simulink model "IMUdataFinalr2PDs"  (R2024a)
settings: Solver=FixedStepAuto  StartTime=0.0  StopTime=100  FixedStep=.01  RelTol=1e-3  EnableMultiTasking=on
undefined symbols (not defined in the file or in its folder): CR, LF
libraries: slpidlib x3, instrumentseriallib x3, hdlsllib x1
settings Model: ExtModeTrigDuration=2  Creator=juanandrespelaezb  LastModifiedBy=Spencer
settings SolverCC: AutoInsertRateTranBlk=on
settings OptimizationCC: EnhancedBackFolding=on  PassReuseOutputArgsThreshold=0  MaxStackSize=64  OptimizeBlockOrder=speed  DifferentSizesBufferReuse=on  OptimizationCustomize=off
settings DebuggingCC: ParameterTunabilityLossMsg=error
settings HardwareCC: ProdBitPerInt=16  ProdBitPerPointer=16  ProdBitPerSizeT=16  ProdBitPerPtrDiffT=16  ProdLargestAtomicFloat=None  ProdWordSize=8  ProdHWDeviceType=Atmel->AVR  UseEmbeddedCoderFeatures=off  UseSimulinkCoderFeatures=off
settings SFSimCC: MATLABDynamicMemAlloc=off
settings RTWCC: Description=Embedded Coder  SystemTargetFile=ert.tlc  HardwareBoard=Arduino Mega 2560  TemplateMakefile=ert_default_tmf  Toolchain=Arduino AVR  BuildConfiguration=Faster Runs
settings CodeAppCC: ForceParamTrailComments=on  OperatorAnnotations=on
settings ERTTargetCC: ERTCustomFileBanners=off  SupportContinuousTime=on  SupportNonInlinedSFcns=on  RemoveResetFunc=off  SupportVariableSizeSignals=on  ModelStepFunctionPrototypeControlCompliant=off  ExtModeTransport=3  ExtModeStaticAlloc=on  ExtModeAutomaticAllocSize=off  ExtModeStaticAllocSize=2048  ExtModeMexFile=ext_xcp  ExtModeIntrfLevel=Level2 - Open

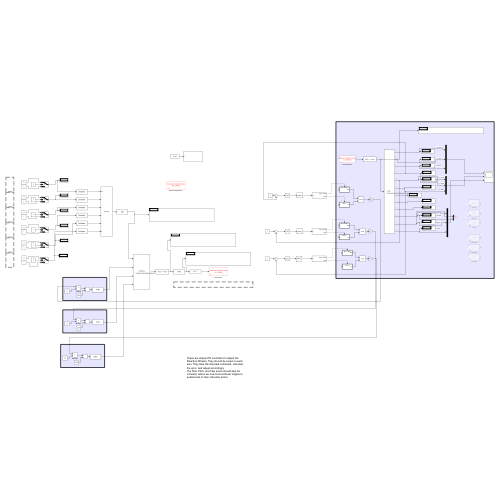
[thumbnail: Simulink's stored preview of the top-level diagram]
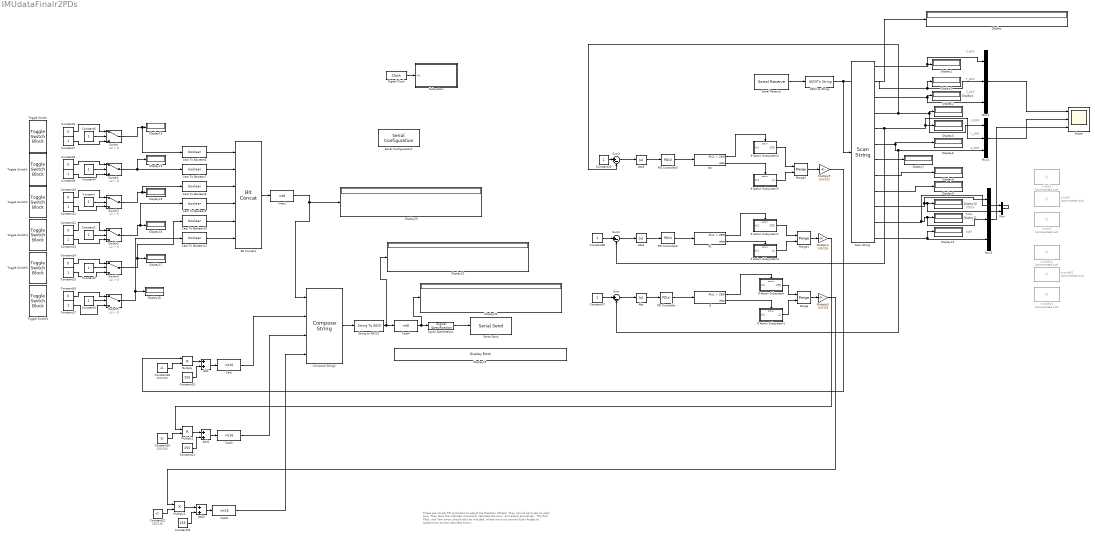
== system IMUdataFinalr2PDs ==
  note: These are simple PD controllers to adjust the Reaction Wheels. They should be tuned on each axis. They take the intended command, calculate the error, and adjust accordingly.
      | The Roll, Pitch, and Yaw errors should also be included, where we must convert Euler Angles to quaternions to then calculate errors.
  note: ROLL
  note: Z_GYR
  note: PITCH
  note: YAW
  note: Y_GYR
  note: X_GYR
  note: Z_ACC
  note: Y_ACC
  note: X_ACC
  ASCII to String : ASCIIToString
  Abs : Abs  SaturateOnIntegerOverflow=off
  Abs2 : Abs  SaturateOnIntegerOverflow=off
  Abs3 : Abs  SaturateOnIntegerOverflow=off
  Add : Sum
  Add1 : Sum
  Add2 : Sum
  Bit Concat1 : hdlsllib/Logic and Bit Operations/Bit Concat  numInputs=6
  Cast : DataTypeConversion  OutDataTypeStr=int16  SaturateOnIntegerOverflow=off  RndMeth=Floor
  Cast To Boolean{6..11} (6 alike) : DataTypeConversion  OutDataTypeStr=boolean  SaturateOnIntegerOverflow=off  RndMeth=Floor
  Cast1 : DataTypeConversion  OutDataTypeStr=int8  SaturateOnIntegerOverflow=off  RndMeth=Floor
  Cast2 : DataTypeConversion  OutDataTypeStr=int16  SaturateOnIntegerOverflow=off  RndMeth=Floor
  Cast3 : DataTypeConversion  OutDataTypeStr=int16  SaturateOnIntegerOverflow=off  RndMeth=Floor
  Cast4 : DataTypeConversion  OutDataTypeStr=int8  SaturateOnIntegerOverflow=off  RndMeth=Floor
  Compose String1 : ComposeString  Format="\"%02d;%03d;%03d;%03d\\n\""
  Constant{,1..5,7,9,11,13,15,17,27..29} (15 alike) : Constant
  Constant{6,8,10,12,14,16} (6 alike) : Constant  Value=0
  Constant18 : Constant  Value=255/100
  Constant19 : Constant  Value=255
  Constant20 : Constant  Value=255/100
  Constant21 : Constant  Value=255
  Constant22 : Constant  Value=255/100
  Constant23 : Constant  Value=255
  Digital Clock : DigitalClock
  Display{,1..18,20..22} (22 alike) : Display
  Display19 : DisplayBlock  LabelPosition=Hide  Format=long  Transparency=1
  If : If  IfExpression=u1 > 255
  If Action Subsystem : Subsystem  TreatAsAtomicUnit=on
  If Action Subsystem1 : Subsystem  TreatAsAtomicUnit=on
  If Action Subsystem2 : Subsystem  TreatAsAtomicUnit=on
  If Action Subsystem3 : Subsystem  TreatAsAtomicUnit=on
  If Action Subsystem4 : Subsystem  TreatAsAtomicUnit=on
  If Action Subsystem5 : Subsystem  TreatAsAtomicUnit=on
  If1 : If  IfExpression=u1 > 255
  If2 : If  IfExpression=u1 > 255
  Merge : Merge
  Merge1 : Merge
  Merge2 : Merge
  Multiply : Product
  Multiply1 : Product
  Multiply2 : Product
  Multiply3 : Gain  Gain=100/255
  Multiply4 : Gain  Gain=100/255
  Multiply5 : Gain  Gain=100/255
  Mux : Mux  Inputs=2
  Mux1 : Mux  Inputs=3
  Mux2 : Mux  Inputs=3
  Mux3 : Mux  Inputs=3
  PID Controller : slpidlib/PID Controller  Controller=PD  Form=Parallel  TimeDomain=Continuous-time  UseExternalTs=off  SampleTime=-1  IntegratorMethod=Forward Euler  FilterMethod=Forward Euler  ControllerParametersSource=internal  P=25  I=1  UseKiTs=off  D=5  UseExternalDerivativeSource=off  N=100  UseFilter=on  TunerSelectOption=Transfer Function Based (PID Tuner App)  InitialConditionSource=internal  InitialConditionForIntegrator=0  InitialConditionForFilter=0  DifferentiatorICPrevScaledInput=0  ExternalReset=none  TrackingMode=off  Kt=1  LimitOutput=off  SatLimitsSource=internal  UpperSaturationLimit=inf  LowerSaturationLimit=-inf  LinearizeAsGain=on  AntiWindupMode=none  Kb=1  LimitIntegrator=off  UpperIntegratorSaturationLimit=inf  LowerIntegratorSaturationLimit=-inf  POutMin=[]  POutMax=[]  IOutMin=[]  IOutMax=[]  DOutMin=[]  DOutMax=[]  NOutMin=[]  NOutMax=[]  SumOutMin=[]  SumOutMax=[]  SaturationOutMin=[]  SaturationOutMax=[]  PParamMin=[]  PParamMax=[]  IParamMin=[]  IParamMax=[]  DParamMin=[]  DParamMax=[]  NParamMin=[]  NParamMax=[]  KbParamMin=[]  KbParamMax=[]  KtParamMin=[]  KtParamMax=[]  KbOutMin=[]  KbOutMax=[]  KtOutMin=[]  KtOutMax=[]  IntegratorOutMin=[]  IntegratorOutMax=[]  FilterOutMin=[]  FilterOutMax=[]  SumI1OutMin=[]  SumI1OutMax=[]  SumI2OutMin=[]  SumI2OutMax=[]  SumI3OutMin=[]  SumI3OutMax=[]  SumI4OutMin=[]  SumI4OutMax=[]  SumDOutMin=[]  SumDOutMax=[]  DifferentiatorOutMin=[]  DifferentiatorOutMax=[]  FilterDiffOutCoefMin=[]  FilterDiffOutCoefMax=[]  ReciprocalOutMin=[]  ReciprocalOutMax=[]  SumDenOutMin=[]  SumDenOutMax=[]  SumNumOutMin=[]  SumNumOutMax=[]  DivideOutMin=[]  DivideOutMax=[]  UdiffTsProdOutMin=[]  UdiffTsProdOutMax=[]  NTsProdOutMin=[]  NTsProdOutMax=[]  UintegralTsProdOutMin=[]  UintegralTsProdOutMax=[]  UngainTsProdOutMin=[]  UngainTsProdOutMax=[]  ClampingZeroOutDataTypeStr=Inherit: Inherit via back propagation  ClampingZeroOutMin=[]  ClampingZeroOutMax=[]  FilterDenConstantOutDataTypeStr=Inherit: Inherit via back propagation  FilterDenConstantOutMin=[]  FilterDenConstantOutMax=[]  PCopyOutDataTypeStr=Inherit: Inherit via back propagation  PCopyOutMin=[]  PCopyOutMax=[]  NCopyOutDataTypeStr=Inherit: Inherit via back propagation  NCopyOutMin=[]  NCopyOutMax=[]  IntegratorContinuousStateAttributes=''  IntegratorStateMustResolveToSignalObject=off  IntegratorRTWStateStorageClass=Auto  FilterContinuousStateAttributes=''  FilterStateMustResolveToSignalObject=off  FilterRTWStateStorageClass=Auto  ParallelPVariant=InternalParameters  IdealPVariant=Disabled  IVariant=Disabled  DVariant=InternalParameters  IntegratorVariant=Disabled  SatVariant=Disabled  AWVariant=Disabled  PCopyVariant=Disabled  TRVariant=Disabled  FdbkBlocksVariant=Forward  IdealPFdbkVariant=Disabled  SatFdbkVariant=Disabled  DerivativeFilterVariant=ContFilter  NVariant=InternalParameters  NCopyVariant=Disabled  FilterICVariant=InternalICsFilter  IntegratorICVariant=Disabled  ExternalResetVariant=Disabled  TRSumVariant=Passthrough  SumFdbkVariant=Disabled  SumVariant=Sum_PD  TsampFilterVariant=InternalTs  TsampNgainVariant=Passthrough  TsampIntegralVariant=Disabled_SignalSpec  ExternalSaturationOutDataTypeStr=Inherit: Same as second input  DerivativeSourceVariant=ErrorSignal
  PID Controller2 : slpidlib/PID Controller  Controller=PD  Form=Parallel  TimeDomain=Continuous-time  UseExternalTs=off  SampleTime=-1  IntegratorMethod=Forward Euler  FilterMethod=Forward Euler  ControllerParametersSource=internal  P=25  I=1  UseKiTs=off  D=5  UseExternalDerivativeSource=off  N=100  UseFilter=on  TunerSelectOption=Transfer Function Based (PID Tuner App)  InitialConditionSource=internal  InitialConditionForIntegrator=0  InitialConditionForFilter=0  DifferentiatorICPrevScaledInput=0  ExternalReset=none  TrackingMode=off  Kt=1  LimitOutput=off  SatLimitsSource=internal  UpperSaturationLimit=inf  LowerSaturationLimit=-inf  LinearizeAsGain=on  AntiWindupMode=none  Kb=1  LimitIntegrator=off  UpperIntegratorSaturationLimit=inf  LowerIntegratorSaturationLimit=-inf  POutMin=[]  POutMax=[]  IOutMin=[]  IOutMax=[]  DOutMin=[]  DOutMax=[]  NOutMin=[]  NOutMax=[]  SumOutMin=[]  SumOutMax=[]  SaturationOutMin=[]  SaturationOutMax=[]  PParamMin=[]  PParamMax=[]  IParamMin=[]  IParamMax=[]  DParamMin=[]  DParamMax=[]  NParamMin=[]  NParamMax=[]  KbParamMin=[]  KbParamMax=[]  KtParamMin=[]  KtParamMax=[]  KbOutMin=[]  KbOutMax=[]  KtOutMin=[]  KtOutMax=[]  IntegratorOutMin=[]  IntegratorOutMax=[]  FilterOutMin=[]  FilterOutMax=[]  SumI1OutMin=[]  SumI1OutMax=[]  SumI2OutMin=[]  SumI2OutMax=[]  SumI3OutMin=[]  SumI3OutMax=[]  SumI4OutMin=[]  SumI4OutMax=[]  SumDOutMin=[]  SumDOutMax=[]  DifferentiatorOutMin=[]  DifferentiatorOutMax=[]  FilterDiffOutCoefMin=[]  FilterDiffOutCoefMax=[]  ReciprocalOutMin=[]  ReciprocalOutMax=[]  SumDenOutMin=[]  SumDenOutMax=[]  SumNumOutMin=[]  SumNumOutMax=[]  DivideOutMin=[]  DivideOutMax=[]  UdiffTsProdOutMin=[]  UdiffTsProdOutMax=[]  NTsProdOutMin=[]  NTsProdOutMax=[]  UintegralTsProdOutMin=[]  UintegralTsProdOutMax=[]  UngainTsProdOutMin=[]  UngainTsProdOutMax=[]  ClampingZeroOutDataTypeStr=Inherit: Inherit via back propagation  ClampingZeroOutMin=[]  ClampingZeroOutMax=[]  FilterDenConstantOutDataTypeStr=Inherit: Inherit via back propagation  FilterDenConstantOutMin=[]  FilterDenConstantOutMax=[]  PCopyOutDataTypeStr=Inherit: Inherit via back propagation  PCopyOutMin=[]  PCopyOutMax=[]  NCopyOutDataTypeStr=Inherit: Inherit via back propagation  NCopyOutMin=[]  NCopyOutMax=[]  IntegratorContinuousStateAttributes=''  IntegratorStateMustResolveToSignalObject=off  IntegratorRTWStateStorageClass=Auto  FilterContinuousStateAttributes=''  FilterStateMustResolveToSignalObject=off  FilterRTWStateStorageClass=Auto  ParallelPVariant=InternalParameters  IdealPVariant=Disabled  IVariant=Disabled  DVariant=InternalParameters  IntegratorVariant=Disabled  SatVariant=Disabled  AWVariant=Disabled  PCopyVariant=Disabled  TRVariant=Disabled  FdbkBlocksVariant=Forward  IdealPFdbkVariant=Disabled  SatFdbkVariant=Disabled  DerivativeFilterVariant=ContFilter  NVariant=InternalParameters  NCopyVariant=Disabled  FilterICVariant=InternalICsFilter  IntegratorICVariant=Disabled  ExternalResetVariant=Disabled  TRSumVariant=Passthrough  SumFdbkVariant=Disabled  SumVariant=Sum_PD  TsampFilterVariant=InternalTs  TsampNgainVariant=Passthrough  TsampIntegralVariant=Disabled_SignalSpec  ExternalSaturationOutDataTypeStr=Inherit: Same as second input  DerivativeSourceVariant=ErrorSignal
  PID Controller3 : slpidlib/PID Controller  Controller=PD  Form=Parallel  TimeDomain=Continuous-time  UseExternalTs=off  SampleTime=-1  IntegratorMethod=Forward Euler  FilterMethod=Forward Euler  ControllerParametersSource=internal  P=25  I=1  UseKiTs=off  D=5  UseExternalDerivativeSource=off  N=100  UseFilter=on  TunerSelectOption=Transfer Function Based (PID Tuner App)  InitialConditionSource=internal  InitialConditionForIntegrator=0  InitialConditionForFilter=0  DifferentiatorICPrevScaledInput=0  ExternalReset=none  TrackingMode=off  Kt=1  LimitOutput=off  SatLimitsSource=internal  UpperSaturationLimit=inf  LowerSaturationLimit=-inf  LinearizeAsGain=on  AntiWindupMode=none  Kb=1  LimitIntegrator=off  UpperIntegratorSaturationLimit=inf  LowerIntegratorSaturationLimit=-inf  POutMin=[]  POutMax=[]  IOutMin=[]  IOutMax=[]  DOutMin=[]  DOutMax=[]  NOutMin=[]  NOutMax=[]  SumOutMin=[]  SumOutMax=[]  SaturationOutMin=[]  SaturationOutMax=[]  PParamMin=[]  PParamMax=[]  IParamMin=[]  IParamMax=[]  DParamMin=[]  DParamMax=[]  NParamMin=[]  NParamMax=[]  KbParamMin=[]  KbParamMax=[]  KtParamMin=[]  KtParamMax=[]  KbOutMin=[]  KbOutMax=[]  KtOutMin=[]  KtOutMax=[]  IntegratorOutMin=[]  IntegratorOutMax=[]  FilterOutMin=[]  FilterOutMax=[]  SumI1OutMin=[]  SumI1OutMax=[]  SumI2OutMin=[]  SumI2OutMax=[]  SumI3OutMin=[]  SumI3OutMax=[]  SumI4OutMin=[]  SumI4OutMax=[]  SumDOutMin=[]  SumDOutMax=[]  DifferentiatorOutMin=[]  DifferentiatorOutMax=[]  FilterDiffOutCoefMin=[]  FilterDiffOutCoefMax=[]  ReciprocalOutMin=[]  ReciprocalOutMax=[]  SumDenOutMin=[]  SumDenOutMax=[]  SumNumOutMin=[]  SumNumOutMax=[]  DivideOutMin=[]  DivideOutMax=[]  UdiffTsProdOutMin=[]  UdiffTsProdOutMax=[]  NTsProdOutMin=[]  NTsProdOutMax=[]  UintegralTsProdOutMin=[]  UintegralTsProdOutMax=[]  UngainTsProdOutMin=[]  UngainTsProdOutMax=[]  ClampingZeroOutDataTypeStr=Inherit: Inherit via back propagation  ClampingZeroOutMin=[]  ClampingZeroOutMax=[]  FilterDenConstantOutDataTypeStr=Inherit: Inherit via back propagation  FilterDenConstantOutMin=[]  FilterDenConstantOutMax=[]  PCopyOutDataTypeStr=Inherit: Inherit via back propagation  PCopyOutMin=[]  PCopyOutMax=[]  NCopyOutDataTypeStr=Inherit: Inherit via back propagation  NCopyOutMin=[]  NCopyOutMax=[]  IntegratorContinuousStateAttributes=''  IntegratorStateMustResolveToSignalObject=off  IntegratorRTWStateStorageClass=Auto  FilterContinuousStateAttributes=''  FilterStateMustResolveToSignalObject=off  FilterRTWStateStorageClass=Auto  ParallelPVariant=InternalParameters  IdealPVariant=Disabled  IVariant=Disabled  DVariant=InternalParameters  IntegratorVariant=Disabled  SatVariant=Disabled  AWVariant=Disabled  PCopyVariant=Disabled  TRVariant=Disabled  FdbkBlocksVariant=Forward  IdealPFdbkVariant=Disabled  SatFdbkVariant=Disabled  DerivativeFilterVariant=ContFilter  NVariant=InternalParameters  NCopyVariant=Disabled  FilterICVariant=InternalICsFilter  IntegratorICVariant=Disabled  ExternalResetVariant=Disabled  TRSumVariant=Passthrough  SumFdbkVariant=Disabled  SumVariant=Sum_PD  TsampFilterVariant=InternalTs  TsampNgainVariant=Passthrough  TsampIntegralVariant=Disabled_SignalSpec  ExternalSaturationOutDataTypeStr=Inherit: Same as second input  DerivativeSourceVariant=ErrorSignal
  Scan String : ScanString  Format="\"%f,%f,%f,%f,%f,%f,%f,%f,%f,%f,%f,%f\""
  Scope : Scope  NumInputPorts=3
  Serial Configuration1 : instrumentseriallib/Serial Configuration  Priority=-200000  PortSel=/dev/cu.usbmodem2101  Port=/dev/cu.usbmodem2101  ComPort=/dev/cu.usbmodem2101  BaudRate=9600  DataBits=8  Parity=none  StopBits=1  ByteOrder=little-endian  FlowControl=none  Timeout=10  SimulateUsing=Interpreted execution  BlockInModel=on  aMode=1
  Serial Receive : instrumentseriallib/Serial Receive  PortSel=/dev/cu.usbmodem2101  Port=/dev/cu.usbmodem2101  ComPort=/dev/cu.usbmodem2101  DataType=uint8  SaveDataType=uint8  ToggleHeader=off  Header=[]  ToggleDataSize=on  DataSize=76  ToggleTerminator=on  Terminator=CR/LF ('\r\n')  CustomTerminator=[]  InputFormat=Column major  EnableBlockingMode=on  ActionDataUnavailable=Output last received value  ActionWhenDataUnavailable=Output last received value  CustomValue=300  SampleTime=.01  SimulateUsing=Interpreted execution  BlockInModel=on  aMode=1
  Serial Send : instrumentseriallib/Serial Send  PortSel=/dev/cu.usbmodem2101  Port=/dev/cu.usbmodem2101  ComPort=/dev/cu.usbmodem2101  Header=[]  Terminator=<none>  CustomTerminator=[]  EnableBlockingMode=on  SimulateUsing=Interpreted execution  BlockInModel=on  aMode=1
  Signal Specification : SignalSpecification  SampleTime=.1
      settings: LockScale=on
  String to ASCII1 : StringToASCII  OutputVectorSize=15
  Subsystem : Subsystem
  Sum : Sum  Inputs=|+-
  Sum2 : Sum  Inputs=|+-
  Sum3 : Sum  Inputs=|+-
  Switch{,1..5} (6 alike) : Switch  Criteria=u2 > Threshold  SaturateOnIntegerOverflow=off  InputSameDT=off
  Toggle Switch{,1..5} (6 alike) : ToggleSwitchBlock
      settings: Values={{'Off', 'On'}, [0 1]}
  massBal1 : Constant  Commented=on  Value=0
  massBal2 : Constant  Commented=on  Value=0
  massBal3 : Constant  Commented=on  Value=0
  wheelX : Constant  Commented=on  Value=0
  wheelY : Constant  Commented=on  Value=0
  wheelZ : Constant  Commented=on  Value=0
  wires:
  Mux/1 -> ?
  Scan String/2 -> Display3/1, Mux1/2
  ASCII to String/1 -> Display/1, Scan String/1
  Scan String/7 -> Display7/1
  Scan String/1 -> Mux1/1, Display1/1
  Mux2/1 -> Scope/2
  Scan String/11 -> Mux/1, Mux3/2, Display11/1
  Mux1/1 -> Scope/1
  Scan String/6 -> Display6/1, Sum/2, Mux2/3
  Scan String/3 -> Display4/1, Mux1/3
  Scan String/5 -> Mux2/2, Display5/1, Sum2/2
  Scan String/8 -> Display8/1
  Scan String/4 -> Display2/1, Mux2/1, Sum3/2
  Scan String/9 -> Display9/1
  Scan String/12 -> Display12/1, Mux3/3
  Scan String/10 -> Mux3/1, Mux/2, Display10/1
  Digital Clock/1 -> Subsystem/1(In1)
  Serial Receive/1 -> ASCII to String/1
  Constant6/1 -> Switch/1
  Constant7/1 -> Switch/3
  Constant8/1 -> Switch1/1
  Constant9/1 -> Switch1/3
  Constant10/1 -> Switch2/1
  Constant11/1 -> Switch2/3
  Constant13/1 -> Switch3/3
  Constant12/1 -> Switch3/1
  Constant14/1 -> Switch4/1
  Constant15/1 -> Switch4/3
  Constant16/1 -> Switch5/1
  Constant17/1 -> Switch5/3
  Constant/1 -> Switch2/2
  Constant1/1 -> Switch3/2
  Constant2/1 -> Switch4/2
  Constant3/1 -> Switch5/2
  Constant4/1 -> Switch1/2
  Constant5/1 -> Switch/2
  Switch/1 -> Cast To Boolean6/1, Display13/1
  Switch1/1 -> Cast To Boolean7/1, Display14/1
  Switch2/1 -> Cast To Boolean8/1, Display15/1
  Switch3/1 -> Cast To Boolean9/1, Display16/1
  Switch4/1 -> Cast To Boolean10/1, Display17/1
  Switch5/1 -> Cast To Boolean11/1, Display18/1
  Cast To Boolean9/1 -> Bit Concat1/4
  Cast To Boolean7/1 -> Bit Concat1/2
  Cast To Boolean10/1 -> Bit Concat1/5
  Cast To Boolean6/1 -> Bit Concat1/1
  Cast To Boolean8/1 -> Bit Concat1/3
  Cast To Boolean11/1 -> Bit Concat1/6
  Bit Concat1/1 -> Cast1/1
  Cast1/1 -> Display20/1, Compose String1/1
  Cast2/1 -> Compose String1/3
  Constant21/1 -> Add1/2
  Constant19/1 -> Add/2
  Constant20/1 -> Multiply1/2
  Multiply1/1 -> Add1/1
  Constant18/1 -> Multiply/2
  Constant23/1 -> Add2/2
  Cast/1 -> Compose String1/2
  Add1/1 -> Cast2/1
  Cast3/1 -> Compose String1/4
  Add/1 -> Cast/1
  Multiply/1 -> Add/1
  Add2/1 -> Cast3/1
  Multiply2/1 -> Add2/1
  Constant22/1 -> Multiply2/2
  Multiply4/1 -> Multiply1/1
  Multiply5/1 -> Multiply/1
  Compose String1/1 -> String to ASCII1/1
  String to ASCII1/1 -> Display21/1, Cast4/1
  Cast4/1 -> Display22/1, Signal Specification/1
  Signal Specification/1 -> Serial Send/1
  Mux3/1 -> Scope/3
  Constant27/1 -> Sum/1
  If Action Subsystem1/1(u1) -> Merge/2
  If Action Subsystem/1(255) -> Merge/1
  Multiply3/1 -> Multiply2/1
  Merge/1 -> Multiply3/1
  If/2 -> If Action Subsystem1/Action
  If/1 -> If Action Subsystem/Action
  Sum/1 -> Abs/1
  Abs/1 -> PID Controller/1
  If1/1 -> If Action Subsystem2/Action
  If Action Subsystem2/1(255) -> Merge1/1
  If1/2 -> If Action Subsystem3/Action
  If Action Subsystem3/1(u1) -> Merge1/2
  Merge1/1 -> Multiply4/1
  Constant28/1 -> Sum2/1
  Abs2/1 -> PID Controller2/1
  PID Controller2/1 -> If1/1
  Sum2/1 -> Abs2/1
  Constant29/1 -> Sum3/1
  PID Controller3/1 -> If2/1
  If2/2 -> If Action Subsystem5/Action
  Abs3/1 -> PID Controller3/1
  If2/1 -> If Action Subsystem4/Action
  Sum3/1 -> Abs3/1
  Merge2/1 -> Multiply5/1
  If Action Subsystem5/1(u1) -> Merge2/2
  If Action Subsystem4/1(255) -> Merge2/1
  PID Controller/1 -> If/1

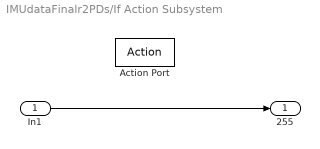
== system IMUdataFinalr2PDs/If Action Subsystem ==
  In1 : Inport
  Action Port : ActionPort  ActionPortLabel=if(u1 > 255)
  255 : Outport
  wires:
  In1/1 -> 255/1

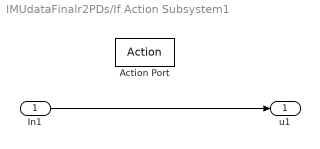
== system IMUdataFinalr2PDs/If Action Subsystem1 ==
  In1 : Inport
  Action Port : ActionPort  ActionPortLabel=else
  u1 : Outport
  wires:
  In1/1 -> u1/1

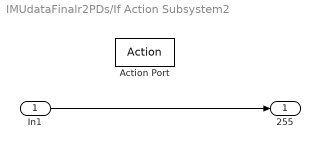
== system IMUdataFinalr2PDs/If Action Subsystem2 ==
  In1 : Inport
  Action Port : ActionPort  ActionPortLabel=if(u1 > 255)
  255 : Outport
  wires:
  In1/1 -> 255/1

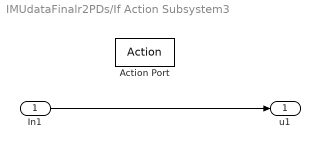
== system IMUdataFinalr2PDs/If Action Subsystem3 ==
  In1 : Inport
  Action Port : ActionPort  ActionPortLabel=else
  u1 : Outport
  wires:
  In1/1 -> u1/1

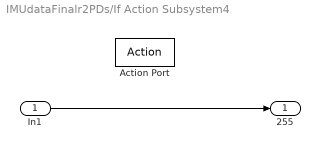
== system IMUdataFinalr2PDs/If Action Subsystem4 ==
  In1 : Inport
  Action Port : ActionPort  ActionPortLabel=if(u1 > 255)
  255 : Outport
  wires:
  In1/1 -> 255/1

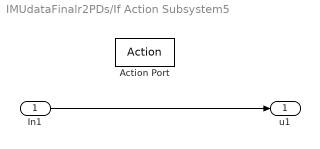
== system IMUdataFinalr2PDs/If Action Subsystem5 ==
  In1 : Inport
  Action Port : ActionPort  ActionPortLabel=else
  u1 : Outport
  wires:
  In1/1 -> u1/1

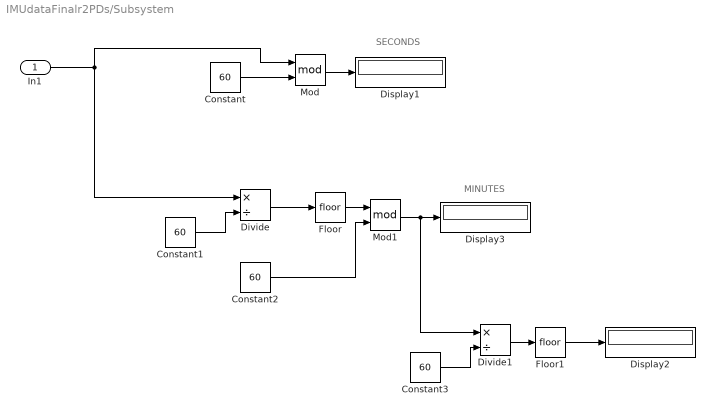
== system IMUdataFinalr2PDs/Subsystem ==
  note: SECONDS
  note: MINUTES
  In1 : Inport
  Constant{,1..3} (4 alike) : Constant  Value=60
  Display1 : Display
  Display2 : Display
  Display3 : Display
  Divide : Product  Inputs=*/
  Divide1 : Product  Inputs=*/
  Floor : Rounding
  Floor1 : Rounding
  Mod : Math  Operator=mod  SignedPower=on
  Mod1 : Math  Operator=mod  SignedPower=on
  wires:
  Constant/1 -> Mod/2
  Mod/1 -> Display1/1
  In1/1 -> Divide/1, Mod/1
  Constant1/1 -> Divide/2
  Divide/1 -> Floor/1
  Floor/1 -> Mod1/1
  Constant2/1 -> Mod1/2
  Mod1/1 -> Divide1/1, Display3/1
  Constant3/1 -> Divide1/2
  Divide1/1 -> Floor1/1
  Floor1/1 -> Display2/1
